simulink subsystem "ContactorsController"  (R2023b)
settings: Solver=VariableStepAuto  StartTime=0.0  StopTime=10.0  RelTol=1e-3
undefined symbols (not defined in the file): tCloseContDelay, tSimCont
settings Model: DataDictionary=Contactors_data.sldd  EnableAccessToBaseWorkspace=off  Creator=Elio  LastModifiedBy=Elio

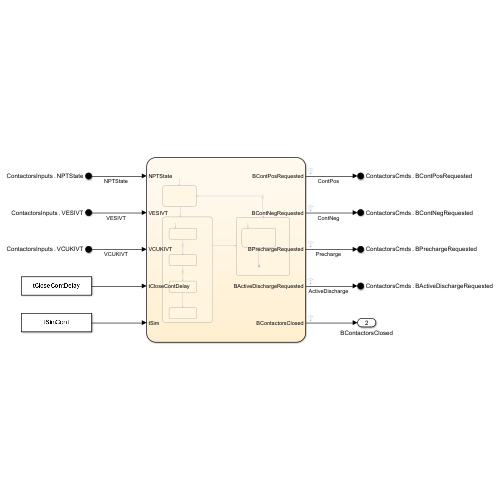
[thumbnail: Simulink's stored preview of the top-level diagram]
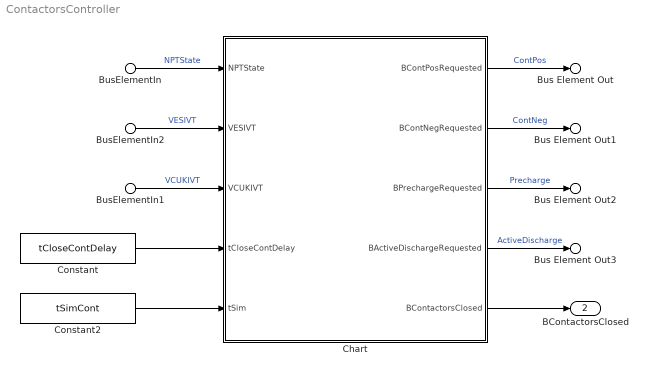
== system ContactorsController ==
  BusElementIn2 : Inport  PortName=ContactorsInputs  Element=VESIVT
  BusElementIn1 : Inport  PortName=ContactorsInputs  Element=VCUKIVT
  BusElementIn : Inport  PortName=ContactorsInputs  Element=NPTState
  Chart : Stateflow chart  TreatAsAtomicUnit=on
      settings: PortSchema="{\"entries\":[{\"content\":{\"sides\":[{\"content\":{\"connectorIds\":[\"In1\",\"In5\",\"In4\",\"In2\",\"In3\"]},\"type\":\"ConnectorPlacement.EquallySpacedRectSide\",\"uuid\":\"5a0065c0-5db5-4462-bbdd-2fd5e45287aa\"},{\"content\":{\"connectorIds\":[\"Out2\",\"Out3\",\"Out1\",\"Out4\",\"Out5\"],\"side\":\"RIGHT\"},\"type\":\"ConnectorPlacement.EquallySpacedRectSide\",\"uuid\":\"ede6eff5-c813-4ab8-91a1-3986418acd87\"},{\"content\":{\"side\":\"TOP\"},\"type\":\"ConnectorPlacement.EquallySpacedRectSide\",\"uuid\":\"7d6725e0-16fb-455f-af2a-820d6785b0ed\"}]},\"type\":\"ConnectorPlacement.EquallySpacedConnector\",\"uuid\":\"9151490c-92d8-4c01-9b8a-0e09fae469db\"}],\"packageUris\":[\"http://schema.mathworks.com/mf0/Connector/R2020b\"],\"version\":\"1.0\"}"
  Constant : Constant  Value=tCloseContDelay  SampleTime=tSimCont
  Constant2 : Constant  Value=tSimCont  SampleTime=tSimCont
  Bus Element Out : Outport  PortName=ContactorsCmds  Element=BContPosRequested
  Bus Element Out1 : Outport  PortName=ContactorsCmds  Element=BContNegRequested
  Bus Element Out2 : Outport  PortName=ContactorsCmds  Element=BPrechargeRequested
  Bus Element Out3 : Outport  PortName=ContactorsCmds  Element=BActiveDischargeRequested
  BContactorsClosed : Outport  Port=2
  wires:
  Chart/5(BContactorsClosed) -> BContactorsClosed/1
  Constant/1 -> Chart/2(tCloseContDelay)
  BusElementIn2/1 -> Chart/5(VESIVT)  "VESIVT"
  BusElementIn/1 -> Chart/1(NPTState)  "NPTState"
  BusElementIn1/1 -> Chart/4(VCUKIVT)  "VCUKIVT"
  Chart/4(BActiveDischargeRequested) -> Bus Element Out3/1  "ActiveDischarge"
  Chart/1(BPrechargeRequested) -> Bus Element Out2/1  "Precharge"
  Chart/3(BContNegRequested) -> Bus Element Out1/1  "ContNeg"
  Chart/2(BContPosRequested) -> Bus Element Out/1  "ContPos"
  Constant2/1 -> Chart/3(tSim)

== stateflow chart ContactorsController/Chart ==
  state STANDBY
    BContPosRequested = 0;
    BContNegRequested = 0;
    BPrechargeRequested = 0;
    BActiveDischargeRequested = 0;
    BContactorsClosed = 0;
    tDelay = 0;
  state CLOSE_SEQUENCE
    state CLOSE_PRECHARGE
      BPrechargeRequested = 1;
    state CLOSE_NEG
      BContNegRequested = 1;
    state CLOSE_POS
      BContPosRequested = 1;
    state OPEN_PRECHARGE
      BPrechargeRequested = 0;
      BContactorsClosed = 1;
    (default) -> CLOSE_PRECHARGE
    CLOSE_PRECHARGE -> (junction 53) : {tDelay += tSim;}
    (junction 53) -> CLOSE_NEG : [tDelay >= tCloseContDelay]
        | {tDelay = 0;}
    CLOSE_NEG -> (junction 57) : {tDelay += tSim;}
    (junction 57) -> CLOSE_POS : [tDelay >= tCloseContDelay]
        | {tDelay = 0;}
    CLOSE_POS -> OPEN_PRECHARGE : [VCUKIVT >= (0.95*VESIVT)]
  state OPEN_SEQUENCE
    state OPEN_CONTACTORS
      BContPosRequested = 0;
      BContNegRequested = 0;
      BPrechargeRequested = 0;
      BActiveDischargeRequested = 1;
    (default) -> OPEN_CONTACTORS
    OPEN_CONTACTORS -> 46 : [VCUKIVT <= 5]
  (default) -> STANDBY
  (junction 28) -> STANDBY
  47 -> (junction 28)
  STANDBY -> CLOSE_SEQUENCE : [NPTState == 1]
  CLOSE_SEQUENCE -> OPEN_SEQUENCE : [NPTState == 4]
      | {tDelay = 0;}
  data: NPTState input; BPrechargeRequested output boolean; BContPosRequested output boolean; BContNegRequested output boolean; BActiveDischargeRequested output boolean; tCloseContDelay input; tDelay local double; tSim input; VCUKIVT input double; VESIVT input double; BContactorsClosed output double
